simulink model "sauna_sim"  (R2023a)
settings: Solver=VariableStepAuto  StartTime=0.0  StopTime=3600*2  RelTol=1e-3  AbsTol=1e-3
undefined symbols (not defined in the file or in its folder): cost_electricity, cost_gas, gebouw2_temp, gebouw_temp, mean_mean, opgiet_deur_d, opgiet_deur_opp, opgiet_muur_1_hout_d, opgiet_muur_1_isol_d, opgiet_muur_1_opp, opgiet_muur_2_opp, opgiet_muur_3_opp, opgiet_muur_4_opp, opgiet_plafond_opp, opgiet_volume, R_hout, R_hout_plafond, R_isol, R_muur_2_gips, R_muur_3_gips, R_muur_3_raam, R_muur_4_buiten, R_muur_4_gips, R_muur_4_raam, R_opgiet_hout, R_opgiet_isol, R_sauna2_deur, R_se, R_si, rho_lucht, sauna1_deur_d, sauna1_deur_opp, sauna1_muur_1_hout_d, sauna1_muur_1_isol_d, sauna1_muur_1_opp, sauna1_muur_2_gips_d, sauna1_muur_2_opp, sauna1_muur_3_gips_d, sauna1_muur_3_opp, sauna1_muur_4_gips_d, sauna1_muur_4_opp, sauna1_plafond_hout_d, sauna1_plafond_isol_d, sauna1_plafond_opp, sauna1_R_muur_2_gips, sauna1_R_muur_3_gips, sauna1_R_muur_4_gips, sauna1_vol, sauna2_deur_opp, sauna2_muur_1_hout_d, sauna2_muur_1_isol_d, sauna2_muur_1_opp, sauna2_muur_2_gips_d, sauna2_muur_2_opp, sauna2_muur_3_gips_d, sauna2_muur_3_opp, sauna2_muur_3_raam_d, sauna2_muur_3_raam_opp, sauna2_muur_4_gips_d, sauna2_muur_4_opp ... (+6)
libraries: fl_lib x491, nesl_utility x30
(part 1 of 6)
settings Model: Creator=thoma  LastModifiedBy=thoma
settings SolverCC: AutoScaleAbsTol=off  AlgebraicLoopSolver=TrustRegion  MaxZcPerStep=1
settings DebuggingCC: UnconnectedInputMsg=warning  UnconnectedOutputMsg=warning  UnconnectedLineMsg=warning  SymbolicDimsDataTypeCodeGenerationDiagnostic=none
settings ModelReferenceCC: EnableRefExpFcnMdlSchedulingChecks=on
settings SFSimCC: CustomCodeUndefinedFunction=UseInterfaceOnly
settings RTWCC: DLArmComputeVersion=19.05
settings SimscapeCC: SimscapeLogType=all  SimscapeLogSimulationStatistics=on  SimscapeLogDataHistory=10000

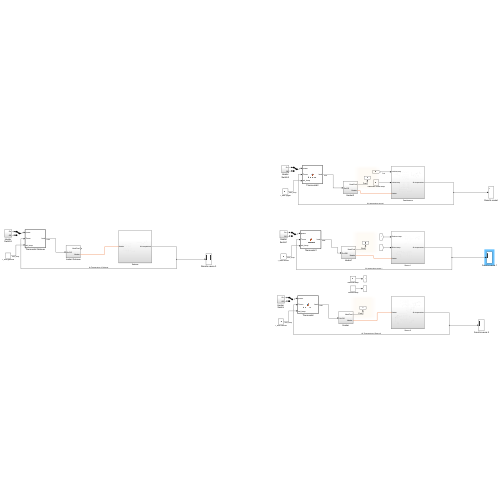
[thumbnail: Simulink's stored preview of the top-level diagram]
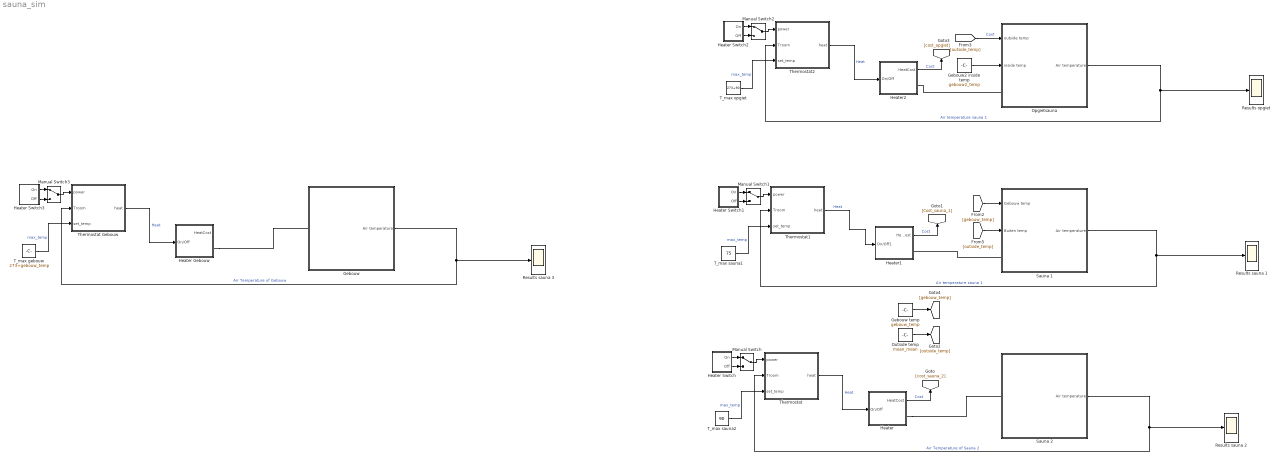
== system sauna_sim ==
  Gebouw : Subsystem
  Gebouw temp : Constant  Value=gebouw_temp
  Gebouw2 inside temp : Constant  Value=gebouw2_temp
  Heater : Subsystem
  Heater Switch : Subsystem
  Heater Switch1 : Subsystem
  Heater Switch2 : Subsystem
  Heater Switch3 : Subsystem
  Heater Gebouw : Subsystem
  Heater1 : Subsystem
  Heater2 : Subsystem
  Manual Switch{,1..3} (4 alike) : ManualSwitch
  Opgietsauna : Subsystem
  Outside temp : Constant  Value=mean_mean
  Results opgiet : Scope
  Results sauna 1 : Scope
  Results sauna 2 : Scope
  Results sauna 3 : Scope
  Sauna 1 : Subsystem
  Sauna 2 : Subsystem
  T_max gebouw : Constant  Value=273+gebouw_temp
  T_max opgiet : Constant  Value=273+90
  T_max sauna1 : Constant  Value=75
  T_max sauna2 : Constant  Value=90
  Thermostat : MATLAB Function  TreatAsAtomicUnit=on
  Thermostat Gebouw : MATLAB Function  TreatAsAtomicUnit=on
  Thermostat1 : MATLAB Function  TreatAsAtomicUnit=on
  Thermostat2 : MATLAB Function  TreatAsAtomicUnit=on
  wires:
  Manual Switch/1 -> Thermostat/1(power)
  Heater Switch/1(On) -> Manual Switch/1
  Heater Switch/2(Off) -> Manual Switch/2
  Thermostat/1(heat) -> Heater/1(On/Off)  "Heat"
  Sauna 2/1(Air temperature) -> Results sauna 2/1, Thermostat/2(Troom)  "Air Temperature of Sauna 2"
  Heater/1(HeatCost) -> [cost_sauna_2]  "Cost"
  T_max sauna2/1 -> Thermostat/3(set_temp)  "max_temp"
  Heater Switch1/1(On) -> Manual Switch1/1
  Heater Switch1/2(Off) -> Manual Switch1/2
  Manual Switch1/1 -> Thermostat1/1(power)
  T_max sauna1/1 -> Thermostat1/3(set_temp)  "max_temp"
  Thermostat1/1(heat) -> Heater1/1(On/Off1)  "Heat"
  Heater1/1(HeatCost) -> [Cost_sauna_1]  "Cost"
  Sauna 1/1(Air temperature) -> Thermostat1/2(Troom), Results sauna 1/1  "Air temperature sauna 1"
  Gebouw2 inside temp/1 -> Opgietsauna/2(inside temp)
  Outside temp/1 -> [outside_temp]
  [outside_temp] -> Opgietsauna/1(outside temp)  "Cost"
  T_max opgiet/1 -> Thermostat2/3(set_temp)  "max_temp"
  Heater2/1(HeatCost) -> [cost_opgiet]  "Cost"
  Manual Switch2/1 -> Thermostat2/1(power)
  Thermostat2/1(heat) -> Heater2/1(On/Off)  "Heat"
  Opgietsauna/1(Air temperature) -> Thermostat2/2(Troom), Results opgiet/1  "Air temperature sauna 1"
  Heater Switch2/1(On) -> Manual Switch2/1
  Heater Switch2/2(Off) -> Manual Switch2/2
  Gebouw temp/1 -> [gebouw_temp]
  [gebouw_temp] -> Sauna 1/1(Gebouw temp)
  [outside_temp] -> Sauna 1/2(Buiten temp)
  Thermostat Gebouw/1(heat) -> Heater Gebouw/1(On/Off)  "Heat"
  Heater Switch3/1(On) -> Manual Switch3/1
  T_max gebouw/1 -> Thermostat Gebouw/3(set_temp)  "max_temp"
  Gebouw/1(Air temperature) -> Results sauna 3/1, Thermostat Gebouw/2(Troom)  "Air Temperature of Gebouw"
  Heater Switch3/2(Off) -> Manual Switch3/2
  Manual Switch3/1 -> Thermostat Gebouw/1(power)
  connections:
  Sauna 1/LConn1 -- Heater1/RConn1
  Opgietsauna/LConn1 -- Heater2/RConn1
  Heater/RConn1 -- Sauna 2/LConn1
  Heater Gebouw/RConn1 -- Gebouw/LConn1

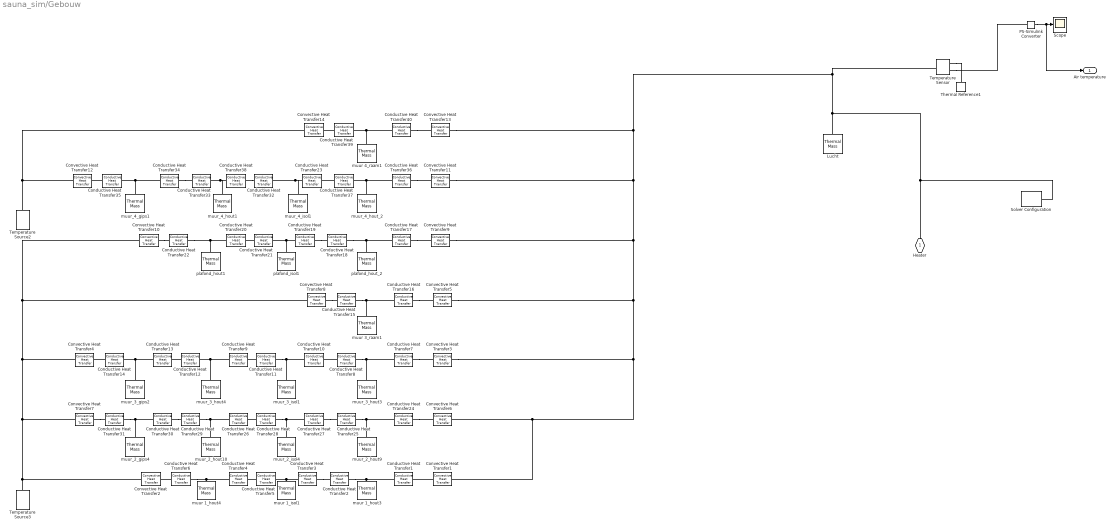
== system sauna_sim/Gebouw ==
  Conductive Heat Transfer{1..2,4,6} (4 alike) : fl_lib/Thermal/Thermal Elements/Conductive Heat Transfer  thermal_type=foundation.enum.ConstantVariableTabulated.Constant  wall_geometry=foundation.enum.ConductionWallGeometry.Planar  area=sauna2_muur_1_opp m^2  thickness=sauna2_muur_1_hout_d/2 m  d_in=0.05 m  d_out=0.1 m  L=1 m  th_cond_min=10 W/(K*m)  th_cond=l_poplar W/(K*m)  th_cond_TLU=[413, 401, 392, 383, 371, 357, 342] W/(K*m)  temp_TLU=[200, 273, 400, 600, 800, 1000, 1200] K  T_specify=off  T_priority=None  T=0 K  T_nominal_specify=off  T_nominal_unit=K  T_nominal_value=1  Q_specify=off  Q_priority=None  Q=0 W  Q_nominal_specify=off  Q_nominal_unit=W  Q_nominal_value=1
  Conductive Heat Transfer10 : fl_lib/Thermal/Thermal Elements/Conductive Heat Transfer  thermal_type=foundation.enum.ConstantVariableTabulated.Constant  wall_geometry=foundation.enum.ConductionWallGeometry.Planar  area=sauna2_muur_3_opp m^2  thickness=sauna2_muur_1_isol_d/2 m  d_in=0.05 m  d_out=0.1 m  L=1 m  th_cond_min=10 W/(K*m)  th_cond=l_isol W/(K*m)  th_cond_TLU=[413, 401, 392, 383, 371, 357, 342] W/(K*m)  temp_TLU=[200, 273, 400, 600, 800, 1000, 1200] K  T_specify=off  T_priority=None  T=0 K  T_nominal_specify=off  T_nominal_unit=K  T_nominal_value=1  Q_specify=off  Q_priority=None  Q=0 W  Q_nominal_specify=off  Q_nominal_unit=W  Q_nominal_value=1
  Conductive Heat Transfer11 : fl_lib/Thermal/Thermal Elements/Conductive Heat Transfer  thermal_type=foundation.enum.ConstantVariableTabulated.Constant  wall_geometry=foundation.enum.ConductionWallGeometry.Planar  area=sauna2_muur_3_opp m^2  thickness=sauna2_muur_1_isol_d/2 m  d_in=0.05 m  d_out=0.1 m  L=1 m  th_cond_min=10 W/(K*m)  th_cond=l_isol W/(K*m)  th_cond_TLU=[413, 401, 392, 383, 371, 357, 342] W/(K*m)  temp_TLU=[200, 273, 400, 600, 800, 1000, 1200] K  T_specify=off  T_priority=None  T=0 K  T_nominal_specify=off  T_nominal_unit=K  T_nominal_value=1  Q_specify=off  Q_priority=None  Q=0 W  Q_nominal_specify=off  Q_nominal_unit=W  Q_nominal_value=1
  Conductive Heat Transfer{7..9,12} (4 alike) : fl_lib/Thermal/Thermal Elements/Conductive Heat Transfer  thermal_type=foundation.enum.ConstantVariableTabulated.Constant  wall_geometry=foundation.enum.ConductionWallGeometry.Planar  area=sauna2_muur_3_opp m^2  thickness=sauna2_muur_1_hout_d/2 m  d_in=0.05 m  d_out=0.1 m  L=1 m  th_cond_min=10 W/(K*m)  th_cond=l_poplar W/(K*m)  th_cond_TLU=[413, 401, 392, 383, 371, 357, 342] W/(K*m)  temp_TLU=[200, 273, 400, 600, 800, 1000, 1200] K  T_specify=off  T_priority=None  T=0 K  T_nominal_specify=off  T_nominal_unit=K  T_nominal_value=1  Q_specify=off  Q_priority=None  Q=0 W  Q_nominal_specify=off  Q_nominal_unit=W  Q_nominal_value=1
  Conductive Heat Transfer13 : fl_lib/Thermal/Thermal Elements/Conductive Heat Transfer  thermal_type=foundation.enum.ConstantVariableTabulated.Constant  wall_geometry=foundation.enum.ConductionWallGeometry.Planar  area=sauna2_muur_3_opp m^2  thickness=sauna2_muur_3_gips_d/2 m  d_in=0.05 m  d_out=0.1 m  L=1 m  th_cond_min=10 W/(K*m)  th_cond=l_gips W/(K*m)  th_cond_TLU=[413, 401, 392, 383, 371, 357, 342] W/(K*m)  temp_TLU=[200, 273, 400, 600, 800, 1000, 1200] K  T_specify=off  T_priority=None  T=0 K  T_nominal_specify=off  T_nominal_unit=K  T_nominal_value=1  Q_specify=off  Q_priority=None  Q=0 W  Q_nominal_specify=off  Q_nominal_unit=W  Q_nominal_value=1
  Conductive Heat Transfer14 : fl_lib/Thermal/Thermal Elements/Conductive Heat Transfer  thermal_type=foundation.enum.ConstantVariableTabulated.Constant  wall_geometry=foundation.enum.ConductionWallGeometry.Planar  area=sauna2_muur_3_opp m^2  thickness=sauna2_muur_3_gips_d/2 m  d_in=0.05 m  d_out=0.1 m  L=1 m  th_cond_min=10 W/(K*m)  th_cond=l_gips W/(K*m)  th_cond_TLU=[413, 401, 392, 383, 371, 357, 342] W/(K*m)  temp_TLU=[200, 273, 400, 600, 800, 1000, 1200] K  T_specify=off  T_priority=None  T=0 K  T_nominal_specify=off  T_nominal_unit=K  T_nominal_value=1  Q_specify=off  Q_priority=None  Q=0 W  Q_nominal_specify=off  Q_nominal_unit=W  Q_nominal_value=1
  Conductive Heat Transfer15 : fl_lib/Thermal/Thermal Elements/Conductive Heat Transfer  thermal_type=foundation.enum.ConstantVariableTabulated.Constant  wall_geometry=foundation.enum.ConductionWallGeometry.Planar  area=sauna2_muur_3_raam_opp m^2  thickness=sauna2_muur_3_raam_d/2 m  d_in=0.05 m  d_out=0.1 m  L=1 m  th_cond_min=10 W/(K*m)  th_cond=l_glas W/(K*m)  th_cond_TLU=[413, 401, 392, 383, 371, 357, 342] W/(K*m)  temp_TLU=[200, 273, 400, 600, 800, 1000, 1200] K  T_specify=off  T_priority=None  T=0 K  T_nominal_specify=off  T_nominal_unit=K  T_nominal_value=1  Q_specify=off  Q_priority=None  Q=0 W  Q_nominal_specify=off  Q_nominal_unit=W  Q_nominal_value=1
  Conductive Heat Transfer16 : fl_lib/Thermal/Thermal Elements/Conductive Heat Transfer  thermal_type=foundation.enum.ConstantVariableTabulated.Constant  wall_geometry=foundation.enum.ConductionWallGeometry.Planar  area=sauna2_muur_3_raam_opp m^2  thickness=sauna2_muur_3_raam_d/2 m  d_in=0.05 m  d_out=0.1 m  L=1 m  th_cond_min=10 W/(K*m)  th_cond=l_glas W/(K*m)  th_cond_TLU=[413, 401, 392, 383, 371, 357, 342] W/(K*m)  temp_TLU=[200, 273, 400, 600, 800, 1000, 1200] K  T_specify=off  T_priority=None  T=0 K  T_nominal_specify=off  T_nominal_unit=K  T_nominal_value=1  Q_specify=off  Q_priority=None  Q=0 W  Q_nominal_specify=off  Q_nominal_unit=W  Q_nominal_value=1
  Conductive Heat Transfer{17..18,20,22} (4 alike) : fl_lib/Thermal/Thermal Elements/Conductive Heat Transfer  thermal_type=foundation.enum.ConstantVariableTabulated.Constant  wall_geometry=foundation.enum.ConductionWallGeometry.Planar  area=sauna2_plafond_opp m^2  thickness=sauna2_plafond_hout_d/2 m  d_in=0.05 m  d_out=0.1 m  L=1 m  th_cond_min=10 W/(K*m)  th_cond=l_poplar W/(K*m)  th_cond_TLU=[413, 401, 392, 383, 371, 357, 342] W/(K*m)  temp_TLU=[200, 273, 400, 600, 800, 1000, 1200] K  T_specify=off  T_priority=None  T=0 K  T_nominal_specify=off  T_nominal_unit=K  T_nominal_value=1  Q_specify=off  Q_priority=None  Q=0 W  Q_nominal_specify=off  Q_nominal_unit=W  Q_nominal_value=1
  Conductive Heat Transfer19 : fl_lib/Thermal/Thermal Elements/Conductive Heat Transfer  thermal_type=foundation.enum.ConstantVariableTabulated.Constant  wall_geometry=foundation.enum.ConductionWallGeometry.Planar  area=sauna2_plafond_opp m^2  thickness=sauna2_plafond_isol_d/2 m  d_in=0.05 m  d_out=0.1 m  L=1 m  th_cond_min=10 W/(K*m)  th_cond=l_isol W/(K*m)  th_cond_TLU=[413, 401, 392, 383, 371, 357, 342] W/(K*m)  temp_TLU=[200, 273, 400, 600, 800, 1000, 1200] K  T_specify=off  T_priority=None  T=0 K  T_nominal_specify=off  T_nominal_unit=K  T_nominal_value=1  Q_specify=off  Q_priority=None  Q=0 W  Q_nominal_specify=off  Q_nominal_unit=W  Q_nominal_value=1
  Conductive Heat Transfer21 : fl_lib/Thermal/Thermal Elements/Conductive Heat Transfer  thermal_type=foundation.enum.ConstantVariableTabulated.Constant  wall_geometry=foundation.enum.ConductionWallGeometry.Planar  area=sauna2_plafond_opp m^2  thickness=sauna2_plafond_isol_d/2 m  d_in=0.05 m  d_out=0.1 m  L=1 m  th_cond_min=10 W/(K*m)  th_cond=l_isol W/(K*m)  th_cond_TLU=[413, 401, 392, 383, 371, 357, 342] W/(K*m)  temp_TLU=[200, 273, 400, 600, 800, 1000, 1200] K  T_specify=off  T_priority=None  T=0 K  T_nominal_specify=off  T_nominal_unit=K  T_nominal_value=1  Q_specify=off  Q_priority=None  Q=0 W  Q_nominal_specify=off  Q_nominal_unit=W  Q_nominal_value=1
  Conductive Heat Transfer23 : fl_lib/Thermal/Thermal Elements/Conductive Heat Transfer  thermal_type=foundation.enum.ConstantVariableTabulated.Constant  wall_geometry=foundation.enum.ConductionWallGeometry.Planar  area=sauna2_muur_4_opp m^2  thickness=sauna2_muur_1_isol_d/2 m  d_in=0.05 m  d_out=0.1 m  L=1 m  th_cond_min=10 W/(K*m)  th_cond=l_isol W/(K*m)  th_cond_TLU=[413, 401, 392, 383, 371, 357, 342] W/(K*m)  temp_TLU=[200, 273, 400, 600, 800, 1000, 1200] K  T_specify=off  T_priority=None  T=0 K  T_nominal_specify=off  T_nominal_unit=K  T_nominal_value=1  Q_specify=off  Q_priority=None  Q=0 W  Q_nominal_specify=off  Q_nominal_unit=W  Q_nominal_value=1
  Conductive Heat Transfer{24..26,29} (4 alike) : fl_lib/Thermal/Thermal Elements/Conductive Heat Transfer  thermal_type=foundation.enum.ConstantVariableTabulated.Constant  wall_geometry=foundation.enum.ConductionWallGeometry.Planar  area=sauna2_muur_2_opp m^2  thickness=sauna2_muur_1_hout_d/2 m  d_in=0.05 m  d_out=0.1 m  L=1 m  th_cond_min=10 W/(K*m)  th_cond=l_poplar W/(K*m)  th_cond_TLU=[413, 401, 392, 383, 371, 357, 342] W/(K*m)  temp_TLU=[200, 273, 400, 600, 800, 1000, 1200] K  T_specify=off  T_priority=None  T=0 K  T_nominal_specify=off  T_nominal_unit=K  T_nominal_value=1  Q_specify=off  Q_priority=None  Q=0 W  Q_nominal_specify=off  Q_nominal_unit=W  Q_nominal_value=1
  Conductive Heat Transfer27 : fl_lib/Thermal/Thermal Elements/Conductive Heat Transfer  thermal_type=foundation.enum.ConstantVariableTabulated.Constant  wall_geometry=foundation.enum.ConductionWallGeometry.Planar  area=sauna2_muur_2_opp m^2  thickness=sauna2_muur_1_isol_d/2 m  d_in=0.05 m  d_out=0.1 m  L=1 m  th_cond_min=10 W/(K*m)  th_cond=l_isol W/(K*m)  th_cond_TLU=[413, 401, 392, 383, 371, 357, 342] W/(K*m)  temp_TLU=[200, 273, 400, 600, 800, 1000, 1200] K  T_specify=off  T_priority=None  T=0 K  T_nominal_specify=off  T_nominal_unit=K  T_nominal_value=1  Q_specify=off  Q_priority=None  Q=0 W  Q_nominal_specify=off  Q_nominal_unit=W  Q_nominal_value=1
  Conductive Heat Transfer28 : fl_lib/Thermal/Thermal Elements/Conductive Heat Transfer  thermal_type=foundation.enum.ConstantVariableTabulated.Constant  wall_geometry=foundation.enum.ConductionWallGeometry.Planar  area=sauna2_muur_2_opp m^2  thickness=sauna2_muur_1_isol_d/2 m  d_in=0.05 m  d_out=0.1 m  L=1 m  th_cond_min=10 W/(K*m)  th_cond=l_isol W/(K*m)  th_cond_TLU=[413, 401, 392, 383, 371, 357, 342] W/(K*m)  temp_TLU=[200, 273, 400, 600, 800, 1000, 1200] K  T_specify=off  T_priority=None  T=0 K  T_nominal_specify=off  T_nominal_unit=K  T_nominal_value=1  Q_specify=off  Q_priority=None  Q=0 W  Q_nominal_specify=off  Q_nominal_unit=W  Q_nominal_value=1
  Conductive Heat Transfer3 : fl_lib/Thermal/Thermal Elements/Conductive Heat Transfer  thermal_type=foundation.enum.ConstantVariableTabulated.Constant  wall_geometry=foundation.enum.ConductionWallGeometry.Planar  area=sauna2_muur_1_opp m^2  thickness=sauna2_muur_1_isol_d/2 m  d_in=0.05 m  d_out=0.1 m  L=1 m  th_cond_min=10 W/(K*m)  th_cond=l_isol W/(K*m)  th_cond_TLU=[413, 401, 392, 383, 371, 357, 342] W/(K*m)  temp_TLU=[200, 273, 400, 600, 800, 1000, 1200] K  T_specify=off  T_priority=None  T=0 K  T_nominal_specify=off  T_nominal_unit=K  T_nominal_value=1  Q_specify=off  Q_priority=None  Q=0 W  Q_nominal_specify=off  Q_nominal_unit=W  Q_nominal_value=1
  Conductive Heat Transfer30 : fl_lib/Thermal/Thermal Elements/Conductive Heat Transfer  thermal_type=foundation.enum.ConstantVariableTabulated.Constant  wall_geometry=foundation.enum.ConductionWallGeometry.Planar  area=sauna2_muur_2_opp m^2  thickness=sauna2_muur_2_gips_d/2 m  d_in=0.05 m  d_out=0.1 m  L=1 m  th_cond_min=10 W/(K*m)  th_cond=l_gips W/(K*m)  th_cond_TLU=[413, 401, 392, 383, 371, 357, 342] W/(K*m)  temp_TLU=[200, 273, 400, 600, 800, 1000, 1200] K  T_specify=off  T_priority=None  T=0 K  T_nominal_specify=off  T_nominal_unit=K  T_nominal_value=1  Q_specify=off  Q_priority=None  Q=0 W  Q_nominal_specify=off  Q_nominal_unit=W  Q_nominal_value=1
  Conductive Heat Transfer31 : fl_lib/Thermal/Thermal Elements/Conductive Heat Transfer  thermal_type=foundation.enum.ConstantVariableTabulated.Constant  wall_geometry=foundation.enum.ConductionWallGeometry.Planar  area=sauna2_muur_2_opp m^2  thickness=sauna2_muur_2_gips_d/2 m  d_in=0.05 m  d_out=0.1 m  L=1 m  th_cond_min=10 W/(K*m)  th_cond=l_gips W/(K*m)  th_cond_TLU=[413, 401, 392, 383, 371, 357, 342] W/(K*m)  temp_TLU=[200, 273, 400, 600, 800, 1000, 1200] K  T_specify=off  T_priority=None  T=0 K  T_nominal_specify=off  T_nominal_unit=K  T_nominal_value=1  Q_specify=off  Q_priority=None  Q=0 W  Q_nominal_specify=off  Q_nominal_unit=W  Q_nominal_value=1
  Conductive Heat Transfer32 : fl_lib/Thermal/Thermal Elements/Conductive Heat Transfer  thermal_type=foundation.enum.ConstantVariableTabulated.Constant  wall_geometry=foundation.enum.ConductionWallGeometry.Planar  area=sauna2_muur_4_opp m^2  thickness=sauna2_muur_1_isol_d/2 m  d_in=0.05 m  d_out=0.1 m  L=1 m  th_cond_min=10 W/(K*m)  th_cond=l_isol W/(K*m)  th_cond_TLU=[413, 401, 392, 383, 371, 357, 342] W/(K*m)  temp_TLU=[200, 273, 400, 600, 800, 1000, 1200] K  T_specify=off  T_priority=None  T=0 K  T_nominal_specify=off  T_nominal_unit=K  T_nominal_value=1  Q_specify=off  Q_priority=None  Q=0 W  Q_nominal_specify=off  Q_nominal_unit=W  Q_nominal_value=1
  Conductive Heat Transfer{33,36..38} (4 alike) : fl_lib/Thermal/Thermal Elements/Conductive Heat Transfer  thermal_type=foundation.enum.ConstantVariableTabulated.Constant  wall_geometry=foundation.enum.ConductionWallGeometry.Planar  area=sauna2_muur_4_opp m^2  thickness=sauna2_muur_1_hout_d/2 m  d_in=0.05 m  d_out=0.1 m  L=1 m  th_cond_min=10 W/(K*m)  th_cond=l_poplar W/(K*m)  th_cond_TLU=[413, 401, 392, 383, 371, 357, 342] W/(K*m)  temp_TLU=[200, 273, 400, 600, 800, 1000, 1200] K  T_specify=off  T_priority=None  T=0 K  T_nominal_specify=off  T_nominal_unit=K  T_nominal_value=1  Q_specify=off  Q_priority=None  Q=0 W  Q_nominal_specify=off  Q_nominal_unit=W  Q_nominal_value=1
  Conductive Heat Transfer34 : fl_lib/Thermal/Thermal Elements/Conductive Heat Transfer  thermal_type=foundation.enum.ConstantVariableTabulated.Constant  wall_geometry=foundation.enum.ConductionWallGeometry.Planar  area=sauna2_muur_4_opp m^2  thickness=sauna2_muur_4_gips_d/2 m  d_in=0.05 m  d_out=0.1 m  L=1 m  th_cond_min=10 W/(K*m)  th_cond=l_gips W/(K*m)  th_cond_TLU=[413, 401, 392, 383, 371, 357, 342] W/(K*m)  temp_TLU=[200, 273, 400, 600, 800, 1000, 1200] K  T_specify=off  T_priority=None  T=0 K  T_nominal_specify=off  T_nominal_unit=K  T_nominal_value=1  Q_specify=off  Q_priority=None  Q=0 W  Q_nominal_specify=off  Q_nominal_unit=W  Q_nominal_value=1
  Conductive Heat Transfer35 : fl_lib/Thermal/Thermal Elements/Conductive Heat Transfer  thermal_type=foundation.enum.ConstantVariableTabulated.Constant  wall_geometry=foundation.enum.ConductionWallGeometry.Planar  area=sauna2_muur_4_opp m^2  thickness=sauna2_muur_4_gips_d/2 m  d_in=0.05 m  d_out=0.1 m  L=1 m  th_cond_min=10 W/(K*m)  th_cond=l_gips W/(K*m)  th_cond_TLU=[413, 401, 392, 383, 371, 357, 342] W/(K*m)  temp_TLU=[200, 273, 400, 600, 800, 1000, 1200] K  T_specify=off  T_priority=None  T=0 K  T_nominal_specify=off  T_nominal_unit=K  T_nominal_value=1  Q_specify=off  Q_priority=None  Q=0 W  Q_nominal_specify=off  Q_nominal_unit=W  Q_nominal_value=1
  Conductive Heat Transfer39 : fl_lib/Thermal/Thermal Elements/Conductive Heat Transfer  thermal_type=foundation.enum.ConstantVariableTabulated.Constant  wall_geometry=foundation.enum.ConductionWallGeometry.Planar  area=sauna2_muur_4_opp m^2  thickness=sauna2_muur_4_raam_d/2 m  d_in=0.05 m  d_out=0.1 m  L=1 m  th_cond_min=10 W/(K*m)  th_cond=sauna2_muur_4_raam_d/R_muur_4_raam W/(K*m)  th_cond_TLU=[413, 401, 392, 383, 371, 357, 342] W/(K*m)  temp_TLU=[200, 273, 400, 600, 800, 1000, 1200] K  T_specify=off  T_priority=None  T=0 K  T_nominal_specify=off  T_nominal_unit=K  T_nominal_value=1  Q_specify=off  Q_priority=None  Q=0 W  Q_nominal_specify=off  Q_nominal_unit=W  Q_nominal_value=1
  Conductive Heat Transfer40 : fl_lib/Thermal/Thermal Elements/Conductive Heat Transfer  thermal_type=foundation.enum.ConstantVariableTabulated.Constant  wall_geometry=foundation.enum.ConductionWallGeometry.Planar  area=sauna2_muur_4_opp m^2  thickness=sauna2_muur_4_raam_d/2 m  d_in=0.05 m  d_out=0.1 m  L=1 m  th_cond_min=10 W/(K*m)  th_cond=sauna2_muur_4_raam_d/R_muur_4_raam W/(K*m)  th_cond_TLU=[413, 401, 392, 383, 371, 357, 342] W/(K*m)  temp_TLU=[200, 273, 400, 600, 800, 1000, 1200] K  T_specify=off  T_priority=None  T=0 K  T_nominal_specify=off  T_nominal_unit=K  T_nominal_value=1  Q_specify=off  Q_priority=None  Q=0 W  Q_nominal_specify=off  Q_nominal_unit=W  Q_nominal_value=1
  Conductive Heat Transfer5 : fl_lib/Thermal/Thermal Elements/Conductive Heat Transfer  thermal_type=foundation.enum.ConstantVariableTabulated.Constant  wall_geometry=foundation.enum.ConductionWallGeometry.Planar  area=sauna2_muur_1_opp m^2  thickness=sauna2_muur_1_isol_d/2 m  d_in=0.05 m  d_out=0.1 m  L=1 m  th_cond_min=10 W/(K*m)  th_cond=l_isol W/(K*m)  th_cond_TLU=[413, 401, 392, 383, 371, 357, 342] W/(K*m)  temp_TLU=[200, 273, 400, 600, 800, 1000, 1200] K  T_specify=off  T_priority=None  T=0 K  T_nominal_specify=off  T_nominal_unit=K  T_nominal_value=1  Q_specify=off  Q_priority=None  Q=0 W  Q_nominal_specify=off  Q_nominal_unit=W  Q_nominal_value=1
  Convective Heat Transfer1 : fl_lib/Thermal/Thermal Elements/Convective Heat Transfer  thermal_type=foundation.enum.constant_variable.constant  area=sauna2_muur_1_opp m^2  heat_tr_coeff=15 W/(K*m^2)  min_heat_tr_coeff=1e-3 W/(K*m^2)  T_specify=off  T_priority=None  T=0 K  T_nominal_specify=off  T_nominal_unit=K  T_nominal_value=1  Q_specify=off  Q_priority=None  Q=0 W  Q_nominal_specify=off  Q_nominal_unit=W  Q_nominal_value=1
  Convective Heat Transfer10 : fl_lib/Thermal/Thermal Elements/Convective Heat Transfer  thermal_type=foundation.enum.constant_variable.constant  area=sauna2_plafond_opp m^2  heat_tr_coeff=15 W/(K*m^2)  min_heat_tr_coeff=1e-3 W/(K*m^2)  T_specify=off  T_priority=None  T=0 K  T_nominal_specify=off  T_nominal_unit=K  T_nominal_value=1  Q_specify=off  Q_priority=None  Q=0 W  Q_nominal_specify=off  Q_nominal_unit=W  Q_nominal_value=1
  Convective Heat Transfer11 : fl_lib/Thermal/Thermal Elements/Convective Heat Transfer  thermal_type=foundation.enum.constant_variable.constant  area=sauna2_muur_4_opp m^2  heat_tr_coeff=15 W/(K*m^2)  min_heat_tr_coeff=1e-3 W/(K*m^2)  T_specify=off  T_priority=None  T=0 K  T_nominal_specify=off  T_nominal_unit=K  T_nominal_value=1  Q_specify=off  Q_priority=None  Q=0 W  Q_nominal_specify=off  Q_nominal_unit=W  Q_nominal_value=1
  Convective Heat Transfer12 : fl_lib/Thermal/Thermal Elements/Convective Heat Transfer  thermal_type=foundation.enum.constant_variable.constant  area=sauna2_muur_4_opp m^2  heat_tr_coeff=30 W/(K*m^2)  min_heat_tr_coeff=1e-3 W/(K*m^2)  T_specify=off  T_priority=None  T=0 K  T_nominal_specify=off  T_nominal_unit=K  T_nominal_value=1  Q_specify=off  Q_priority=None  Q=0 W  Q_nominal_specify=off  Q_nominal_unit=W  Q_nominal_value=1
  Convective Heat Transfer13 : fl_lib/Thermal/Thermal Elements/Convective Heat Transfer  thermal_type=foundation.enum.constant_variable.constant  area=sauna2_muur_4_opp m^2  heat_tr_coeff=15 W/(K*m^2)  min_heat_tr_coeff=1e-3 W/(K*m^2)  T_specify=off  T_priority=None  T=0 K  T_nominal_specify=off  T_nominal_unit=K  T_nominal_value=1  Q_specify=off  Q_priority=None  Q=0 W  Q_nominal_specify=off  Q_nominal_unit=W  Q_nominal_value=1
  Convective Heat Transfer14 : fl_lib/Thermal/Thermal Elements/Convective Heat Transfer  thermal_type=foundation.enum.constant_variable.constant  area=sauna2_muur_4_opp m^2  heat_tr_coeff=30 W/(K*m^2)  min_heat_tr_coeff=1e-3 W/(K*m^2)  T_specify=off  T_priority=None  T=0 K  T_nominal_specify=off  T_nominal_unit=K  T_nominal_value=1  Q_specify=off  Q_priority=None  Q=0 W  Q_nominal_specify=off  Q_nominal_unit=W  Q_nominal_value=1
  Convective Heat Transfer2 : fl_lib/Thermal/Thermal Elements/Convective Heat Transfer  thermal_type=foundation.enum.constant_variable.constant  area=sauna2_muur_1_opp m^2  heat_tr_coeff=15 W/(K*m^2)  min_heat_tr_coeff=1e-3 W/(K*m^2)  T_specify=off  T_priority=None  T=0 K  T_nominal_specify=off  T_nominal_unit=K  T_nominal_value=1  Q_specify=off  Q_priority=None  Q=0 W  Q_nominal_specify=off  Q_nominal_unit=W  Q_nominal_value=1
  Convective Heat Transfer3 : fl_lib/Thermal/Thermal Elements/Convective Heat Transfer  thermal_type=foundation.enum.constant_variable.constant  area=sauna2_muur_3_opp m^2  heat_tr_coeff=15 W/(K*m^2)  min_heat_tr_coeff=1e-3 W/(K*m^2)  T_specify=off  T_priority=None  T=0 K  T_nominal_specify=off  T_nominal_unit=K  T_nominal_value=1  Q_specify=off  Q_priority=None  Q=0 W  Q_nominal_specify=off  Q_nominal_unit=W  Q_nominal_value=1
  Convective Heat Transfer4 : fl_lib/Thermal/Thermal Elements/Convective Heat Transfer  thermal_type=foundation.enum.constant_variable.constant  area=sauna2_muur_3_opp m^2  heat_tr_coeff=15 W/(K*m^2)  min_heat_tr_coeff=1e-3 W/(K*m^2)  T_specify=off  T_priority=None  T=0 K  T_nominal_specify=off  T_nominal_unit=K  T_nominal_value=1  Q_specify=off  Q_priority=None  Q=0 W  Q_nominal_specify=off  Q_nominal_unit=W  Q_nominal_value=1
  Convective Heat Transfer5 : fl_lib/Thermal/Thermal Elements/Convective Heat Transfer  thermal_type=foundation.enum.constant_variable.constant  area=sauna2_muur_3_raam_opp m^2  heat_tr_coeff=15 W/(K*m^2)  min_heat_tr_coeff=1e-3 W/(K*m^2)  T_specify=off  T_priority=None  T=0 K  T_nominal_specify=off  T_nominal_unit=K  T_nominal_value=1  Q_specify=off  Q_priority=None  Q=0 W  Q_nominal_specify=off  Q_nominal_unit=W  Q_nominal_value=1
  Convective Heat Transfer6 : fl_lib/Thermal/Thermal Elements/Convective Heat Transfer  thermal_type=foundation.enum.constant_variable.constant  area=sauna2_muur_2_opp m^2  heat_tr_coeff=15 W/(K*m^2)  min_heat_tr_coeff=1e-3 W/(K*m^2)  T_specify=off  T_priority=None  T=0 K  T_nominal_specify=off  T_nominal_unit=K  T_nominal_value=1  Q_specify=off  Q_priority=None  Q=0 W  Q_nominal_specify=off  Q_nominal_unit=W  Q_nominal_value=1
  Convective Heat Transfer7 : fl_lib/Thermal/Thermal Elements/Convective Heat Transfer  thermal_type=foundation.enum.constant_variable.constant  area=sauna2_muur_2_opp m^2  heat_tr_coeff=15 W/(K*m^2)  min_heat_tr_coeff=1e-3 W/(K*m^2)  T_specify=off  T_priority=None  T=0 K  T_nominal_specify=off  T_nominal_unit=K  T_nominal_value=1  Q_specify=off  Q_priority=None  Q=0 W  Q_nominal_specify=off  Q_nominal_unit=W  Q_nominal_value=1
  Convective Heat Transfer8 : fl_lib/Thermal/Thermal Elements/Convective Heat Transfer  thermal_type=foundation.enum.constant_variable.constant  area=sauna2_muur_3_raam_opp m^2  heat_tr_coeff=15 W/(K*m^2)  min_heat_tr_coeff=1e-3 W/(K*m^2)  T_specify=off  T_priority=None  T=0 K  T_nominal_specify=off  T_nominal_unit=K  T_nominal_value=1  Q_specify=off  Q_priority=None  Q=0 W  Q_nominal_specify=off  Q_nominal_unit=W  Q_nominal_value=1
  Convective Heat Transfer9 : fl_lib/Thermal/Thermal Elements/Convective Heat Transfer  thermal_type=foundation.enum.constant_variable.constant  area=sauna2_plafond_opp m^2  heat_tr_coeff=15 W/(K*m^2)  min_heat_tr_coeff=1e-3 W/(K*m^2)  T_specify=off  T_priority=None  T=0 K  T_nominal_specify=off  T_nominal_unit=K  T_nominal_value=1  Q_specify=off  Q_priority=None  Q=0 W  Q_nominal_specify=off  Q_nominal_unit=W  Q_nominal_value=1
  Lucht : fl_lib/Thermal/Thermal Elements/Thermal Mass  mass_type=foundation.enum.constant_variable.constant  mass=sauna2_vol*rho_lucht kg  sp_heat=cp_lucht J/(K*kg)  mass_min=1e-6 kg  num_ports=foundation.enum.numPorts2.one  m_specify=off  m_priority=High  m=1 kg  m_nominal_specify=off  m_nominal_unit=kg  m_nominal_value=1  T_specify=on  T_priority=High  T=300 K  T_nominal_specify=off  T_nominal_unit=K  T_nominal_value=1  Q_specify=off  Q_priority=None  Q=0 W  Q_nominal_specify=off  Q_nominal_unit=W  Q_nominal_value=1
  PS-Simulink Converter : nesl_utility/PS-Simulink Converter  PhysicalDomain=network_engine_domain  SubClassName=ps_output  LeftPortType=input  RightPortType=output  PseudoPeriodic=off  Frequencies=[]  VectorFormat=1-D array  Unit=degC  AffineConversion=on
  Scope : Scope
  Solver Configuration : nesl_utility/Solver Configuration  PhysicalDomain=network_engine_domain  SubClassName=solver  LeftPortType=input  RightPortType=generic  Tones=[]  Harmonics=[]  SimulateNoise=off  Profile=off  UseLocalSampling=off  EnableSwitchedLinearOptims=on  FrequencyDomain=off  UseCCode=off  RelTol=0.001  AbsTol=1e-06  MinStep=1e-09  ToWorkspace=off  RevertToSquareIcSolve=off  NumHomotopyIterations=100  PhasorMode=off  PhasorModeNumHarmonics=1  ConsistencySolver=NEWTON_XTOL_AFTER_FTOL  IndexReductionMethod=DerivativeReplacement  DoDC=off  ResidualTolerance=1e-09  ConsistencyTolSource=GLOBAL  ConsistencyAbsTol=0.001  ConsistencyRelTol=0.001  ConsistencyTolFactor=0.001  UseLocalSolver=off  LocalSolverChoice=NE_BACKWARD_EULER_ADVANCER  ResolveIndetEquations=on  FunctionEvalNumThread=1  LocalSolverSampleTime=0.001  DoFixedCost=off  MaxNonlinIter=3  MaxModeIter=2  ComputeImpulses=off  ImpulseIterations=2  LinearAlgebra=auto  LinearAlgebraNumThread=0  EquationFormulation=NE_TIME_EF  DelaysMemoryBudget=1024  AutomaticFiltering=on  FilteringTimeConstant=0.001  PartitionStorageMethod=AS_NEEDED  PartitionMemoryBudget=1024  PartitionMethod=ROBUST
  Temperature Sensor : fl_lib/Thermal/Thermal Sensors/Temperature Sensor  temperature_measure=foundation.enum.MeasurementReference.difference
  Temperature Source2 : fl_lib/Thermal/Thermal Sources/Temperature Source  temperature=mean_mean+273 K
  Temperature Source3 : fl_lib/Thermal/Thermal Sources/Temperature Source  temperature=gebouw_temp+273 K
  Thermal Reference1 : fl_lib/Thermal/Thermal Elements/Thermal Reference
  muur 1_hout3 : fl_lib/Thermal/Thermal Elements/Thermal Mass  mass_type=foundation.enum.constant_variable.constant  mass=sauna2_muur_1_hout_1_m kg  sp_heat=cp_poplar J/(K*kg)  mass_min=1e-6 kg  num_ports=foundation.enum.numPorts2.one  m_specify=off  m_priority=High  m=1 kg  m_nominal_specify=off  m_nominal_unit=kg  m_nominal_value=1  T_specify=off  T_priority=High  T=300 K  T_nominal_specify=off  T_nominal_unit=K  T_nominal_value=1  Q_specify=off  Q_priority=None  Q=0 W  Q_nominal_specify=off  Q_nominal_unit=W  Q_nominal_value=1
  muur 1_hout4 : fl_lib/Thermal/Thermal Elements/Thermal Mass  mass_type=foundation.enum.constant_variable.constant  mass=sauna2_muur_1_hout_2_m kg  sp_heat=cp_poplar J/(K*kg)  mass_min=1e-6 kg  num_ports=foundation.enum.numPorts2.one  m_specify=off  m_priority=High  m=1 kg  m_nominal_specify=off  m_nominal_unit=kg  m_nominal_value=1  T_specify=off  T_priority=High  T=300 K  T_nominal_specify=off  T_nominal_unit=K  T_nominal_value=1  Q_specify=off  Q_priority=None  Q=0 W  Q_nominal_specify=off  Q_nominal_unit=W  Q_nominal_value=1
  muur 1_isol1 : fl_lib/Thermal/Thermal Elements/Thermal Mass  mass_type=foundation.enum.constant_variable.constant  mass=sauna2_muur_1_isol_m kg  sp_heat=cp_isol J/(K*kg)  mass_min=1e-6 kg  num_ports=foundation.enum.numPorts2.one  m_specify=off  m_priority=High  m=1 kg  m_nominal_specify=off  m_nominal_unit=kg  m_nominal_value=1  T_specify=off  T_priority=High  T=300 K  T_nominal_specify=off  T_nominal_unit=K  T_nominal_value=1  Q_specify=off  Q_priority=None  Q=0 W  Q_nominal_specify=off  Q_nominal_unit=W  Q_nominal_value=1
  muur 3_raam1 : fl_lib/Thermal/Thermal Elements/Thermal Mass  mass_type=foundation.enum.constant_variable.constant  mass=sauna2_muur_3_raam_m kg  sp_heat=cp_glas J/(K*kg)  mass_min=1e-6 kg  num_ports=foundation.enum.numPorts2.one  m_specify=off  m_priority=High  m=1 kg  m_nominal_specify=off  m_nominal_unit=kg  m_nominal_value=1  T_specify=off  T_priority=High  T=300 K  T_nominal_specify=off  T_nominal_unit=K  T_nominal_value=1  Q_specify=off  Q_priority=None  Q=0 W  Q_nominal_specify=off  Q_nominal_unit=W  Q_nominal_value=1
  muur 4_raam1 : fl_lib/Thermal/Thermal Elements/Thermal Mass  mass_type=foundation.enum.constant_variable.constant  mass=sauna2_muur_4_raam_m kg  sp_heat=cp_glas J/(K*kg)  mass_min=1e-6 kg  num_ports=foundation.enum.numPorts2.one  m_specify=off  m_priority=High  m=1 kg  m_nominal_specify=off  m_nominal_unit=kg  m_nominal_value=1  T_specify=off  T_priority=High  T=300 K  T_nominal_specify=off  T_nominal_unit=K  T_nominal_value=1  Q_specify=off  Q_priority=None  Q=0 W  Q_nominal_specify=off  Q_nominal_unit=W  Q_nominal_value=1
  muur_2_gips4 : fl_lib/Thermal/Thermal Elements/Thermal Mass  mass_type=foundation.enum.constant_variable.constant  mass=sauna2_muur_2_gips_m kg  sp_heat=cp_gips J/(K*kg)  mass_min=1e-6 kg  num_ports=foundation.enum.numPorts2.one  m_specify=off  m_priority=High  m=1 kg  m_nominal_specify=off  m_nominal_unit=kg  m_nominal_value=1  T_specify=off  T_priority=High  T=300 K  T_nominal_specify=off  T_nominal_unit=K  T_nominal_value=1  Q_specify=off  Q_priority=None  Q=0 W  Q_nominal_specify=off  Q_nominal_unit=W  Q_nominal_value=1
  muur_2_hout10 : fl_lib/Thermal/Thermal Elements/Thermal Mass  mass_type=foundation.enum.constant_variable.constant  mass=sauna2_muur_2_hout_1_m kg  sp_heat=cp_poplar J/(K*kg)  mass_min=1e-6 kg  num_ports=foundation.enum.numPorts2.one  m_specify=off  m_priority=High  m=1 kg  m_nominal_specify=off  m_nominal_unit=kg  m_nominal_value=1  T_specify=off  T_priority=High  T=300 K  T_nominal_specify=off  T_nominal_unit=K  T_nominal_value=1  Q_specify=off  Q_priority=None  Q=0 W  Q_nominal_specify=off  Q_nominal_unit=W  Q_nominal_value=1
  muur_2_hout9 : fl_lib/Thermal/Thermal Elements/Thermal Mass  mass_type=foundation.enum.constant_variable.constant  mass=sauna2_muur_2_hout_1_m kg  sp_heat=cp_poplar J/(K*kg)  mass_min=1e-6 kg  num_ports=foundation.enum.numPorts2.one  m_specify=off  m_priority=High  m=1 kg  m_nominal_specify=off  m_nominal_unit=kg  m_nominal_value=1  T_specify=off  T_priority=High  T=300 K  T_nominal_specify=off  T_nominal_unit=K  T_nominal_value=1  Q_specify=off  Q_priority=None  Q=0 W  Q_nominal_specify=off  Q_nominal_unit=W  Q_nominal_value=1
  muur_2_isol4 : fl_lib/Thermal/Thermal Elements/Thermal Mass  mass_type=foundation.enum.constant_variable.constant  mass=sauna2_muur_2_isol_m kg  sp_heat=cp_isol J/(K*kg)  mass_min=1e-6 kg  num_ports=foundation.enum.numPorts2.one  m_specify=off  m_priority=High  m=1 kg  m_nominal_specify=off  m_nominal_unit=kg  m_nominal_value=1  T_specify=off  T_priority=High  T=300 K  T_nominal_specify=off  T_nominal_unit=K  T_nominal_value=1  Q_specify=off  Q_priority=None  Q=0 W  Q_nominal_specify=off  Q_nominal_unit=W  Q_nominal_value=1
  muur_3_gips2 : fl_lib/Thermal/Thermal Elements/Thermal Mass  mass_type=foundation.enum.constant_variable.constant  mass=sauna2_muur_3_gips_m kg  sp_heat=cp_gips J/(K*kg)  mass_min=1e-6 kg  num_ports=foundation.enum.numPorts2.one  m_specify=off  m_priority=High  m=1 kg  m_nominal_specify=off  m_nominal_unit=kg  m_nominal_value=1  T_specify=off  T_priority=High  T=300 K  T_nominal_specify=off  T_nominal_unit=K  T_nominal_value=1  Q_specify=off  Q_priority=None  Q=0 W  Q_nominal_specify=off  Q_nominal_unit=W  Q_nominal_value=1
  muur_3_hout3 : fl_lib/Thermal/Thermal Elements/Thermal Mass  mass_type=foundation.enum.constant_variable.constant  mass=sauna2_muur_3_hout_1_m kg  sp_heat=cp_poplar J/(K*kg)  mass_min=1e-6 kg  num_ports=foundation.enum.numPorts2.one  m_specify=off  m_priority=High  m=1 kg  m_nominal_specify=off  m_nominal_unit=kg  m_nominal_value=1  T_specify=off  T_priority=High  T=300 K  T_nominal_specify=off  T_nominal_unit=K  T_nominal_value=1  Q_specify=off  Q_priority=None  Q=0 W  Q_nominal_specify=off  Q_nominal_unit=W  Q_nominal_value=1
  muur_3_hout4 : fl_lib/Thermal/Thermal Elements/Thermal Mass  mass_type=foundation.enum.constant_variable.constant  mass=sauna2_muur_3_hout_2_m kg  sp_heat=cp_poplar J/(K*kg)  mass_min=1e-6 kg  num_ports=foundation.enum.numPorts2.one  m_specify=off  m_priority=High  m=1 kg  m_nominal_specify=off  m_nominal_unit=kg  m_nominal_value=1  T_specify=off  T_priority=High  T=300 K  T_nominal_specify=off  T_nominal_unit=K  T_nominal_value=1  Q_specify=off  Q_priority=None  Q=0 W  Q_nominal_specify=off  Q_nominal_unit=W  Q_nominal_value=1
  muur_3_isol1 : fl_lib/Thermal/Thermal Elements/Thermal Mass  mass_type=foundation.enum.constant_variable.constant  mass=sauna2_muur_3_isol_m kg  sp_heat=cp_isol J/(K*kg)  mass_min=1e-6 kg  num_ports=foundation.enum.numPorts2.one  m_specify=off  m_priority=High  m=1 kg  m_nominal_specify=off  m_nominal_unit=kg  m_nominal_value=1  T_specify=off  T_priority=High  T=300 K  T_nominal_specify=off  T_nominal_unit=K  T_nominal_value=1  Q_specify=off  Q_priority=None  Q=0 W  Q_nominal_specify=off  Q_nominal_unit=W  Q_nominal_value=1
  muur_4_gips1 : fl_lib/Thermal/Thermal Elements/Thermal Mass  mass_type=foundation.enum.constant_variable.constant  mass=sauna2_muur_4_gips_m kg  sp_heat=cp_gips J/(K*kg)  mass_min=1e-6 kg  num_ports=foundation.enum.numPorts2.one  m_specify=off  m_priority=High  m=1 kg  m_nominal_specify=off  m_nominal_unit=kg  m_nominal_value=1  T_specify=off  T_priority=High  T=300 K  T_nominal_specify=off  T_nominal_unit=K  T_nominal_value=1  Q_specify=off  Q_priority=None  Q=0 W  Q_nominal_specify=off  Q_nominal_unit=W  Q_nominal_value=1
  muur_4_hout1 : fl_lib/Thermal/Thermal Elements/Thermal Mass  mass_type=foundation.enum.constant_variable.constant  mass=sauna2_muur_4_hout_2_m kg  sp_heat=cp_poplar J/(K*kg)  mass_min=1e-6 kg  num_ports=foundation.enum.numPorts2.one  m_specify=off  m_priority=High  m=1 kg  m_nominal_specify=off  m_nominal_unit=kg  m_nominal_value=1  T_specify=off  T_priority=High  T=300 K  T_nominal_specify=off  T_nominal_unit=K  T_nominal_value=1  Q_specify=off  Q_priority=None  Q=0 W  Q_nominal_specify=off  Q_nominal_unit=W  Q_nominal_value=1
  muur_4_hout_2 : fl_lib/Thermal/Thermal Elements/Thermal Mass  mass_type=foundation.enum.constant_variable.constant  mass=sauna2_muur_4_hout_1_m kg  sp_heat=cp_poplar J/(K*kg)  mass_min=1e-6 kg  num_ports=foundation.enum.numPorts2.one  m_specify=off  m_priority=High  m=1 kg  m_nominal_specify=off  m_nominal_unit=kg  m_nominal_value=1  T_specify=off  T_priority=High  T=300 K  T_nominal_specify=off  T_nominal_unit=K  T_nominal_value=1  Q_specify=off  Q_priority=None  Q=0 W  Q_nominal_specify=off  Q_nominal_unit=W  Q_nominal_value=1
  muur_4_isol1 : fl_lib/Thermal/Thermal Elements/Thermal Mass  mass_type=foundation.enum.constant_variable.constant  mass=sauna2_muur_4_isol_m kg  sp_heat=cp_isol J/(K*kg)  mass_min=1e-6 kg  num_ports=foundation.enum.numPorts2.one  m_specify=off  m_priority=High  m=1 kg  m_nominal_specify=off  m_nominal_unit=kg  m_nominal_value=1  T_specify=off  T_priority=High  T=300 K  T_nominal_specify=off  T_nominal_unit=K  T_nominal_value=1  Q_specify=off  Q_priority=None  Q=0 W  Q_nominal_specify=off  Q_nominal_unit=W  Q_nominal_value=1
  plafond_hout1 : fl_lib/Thermal/Thermal Elements/Thermal Mass  mass_type=foundation.enum.constant_variable.constant  mass=sauna2_plafond_hout_2_m kg  sp_heat=cp_poplar J/(K*kg)  mass_min=1e-6 kg  num_ports=foundation.enum.numPorts2.one  m_specify=off  m_priority=High  m=1 kg  m_nominal_specify=off  m_nominal_unit=kg  m_nominal_value=1  T_specify=off  T_priority=High  T=300 K  T_nominal_specify=off  T_nominal_unit=K  T_nominal_value=1  Q_specify=off  Q_priority=None  Q=0 W  Q_nominal_specify=off  Q_nominal_unit=W  Q_nominal_value=1
  plafond_hout_2 : fl_lib/Thermal/Thermal Elements/Thermal Mass  mass_type=foundation.enum.constant_variable.constant  mass=sauna2_plafond_hout_1_m kg  sp_heat=cp_poplar J/(K*kg)  mass_min=1e-6 kg  num_ports=foundation.enum.numPorts2.one  m_specify=off  m_priority=High  m=1 kg  m_nominal_specify=off  m_nominal_unit=kg  m_nominal_value=1  T_specify=off  T_priority=High  T=300 K  T_nominal_specify=off  T_nominal_unit=K  T_nominal_value=1  Q_specify=off  Q_priority=None  Q=0 W  Q_nominal_specify=off  Q_nominal_unit=W  Q_nominal_value=1
  plafond_isol1 : fl_lib/Thermal/Thermal Elements/Thermal Mass  mass_type=foundation.enum.constant_variable.constant  mass=sauna2_plafond_isol_m kg  sp_heat=cp_isol J/(K*kg)  mass_min=1e-6 kg  num_ports=foundation.enum.numPorts2.one  m_specify=off  m_priority=High  m=1 kg  m_nominal_specify=off  m_nominal_unit=kg  m_nominal_value=1  T_specify=off  T_priority=High  T=300 K  T_nominal_specify=off  T_nominal_unit=K  T_nominal_value=1  Q_specify=off  Q_priority=None  Q=0 W  Q_nominal_specify=off  Q_nominal_unit=W  Q_nominal_value=1
  Heater : PMIOPort  Tag=PMCPort  Side=Left
  Air temperature : Outport
  wires:
  PS-Simulink Converter/1 -> Air temperature/1, Scope/1
  connections:
  Temperature Sensor/RConn2 -- PS-Simulink Converter/LConn1
  Heater/RConn1 -- Lucht/LConn1 -- Temperature Sensor/LConn1 -- Convective Heat Transfer13/LConn1 -- Convective Heat Transfer3/LConn1 -- Convective Heat Transfer1/LConn1 -- Convective Heat Transfer6/LConn1 -- Convective Heat Transfer5/LConn1 -- Convective Heat Transfer9/LConn1 -- Convective Heat Transfer11/LConn1 -- Solver Configuration/RConn1
  Temperature Sensor/RConn1 -- Thermal Reference1/LConn1
  Conductive Heat Transfer24/RConn1 -- muur_2_hout9/LConn1 -- Conductive Heat Transfer25/LConn1
  Conductive Heat Transfer26/RConn1 -- muur_2_hout10/LConn1 -- Conductive Heat Transfer29/LConn1
  Conductive Heat Transfer27/RConn1 -- muur_2_isol4/LConn1 -- Conductive Heat Transfer28/LConn1
  Conductive Heat Transfer30/RConn1 -- muur_2_gips4/LConn1 -- Conductive Heat Transfer31/LConn1
  Convective Heat Transfer7/LConn1 -- Conductive Heat Transfer31/RConn1
  Conductive Heat Transfer27/LConn1 -- Conductive Heat Transfer25/RConn1
  Conductive Heat Transfer30/LConn1 -- Conductive Heat Transfer29/RConn1
  Conductive Heat Transfer28/RConn1 -- Conductive Heat Transfer26/LConn1
  Conductive Heat Transfer24/LConn1 -- Convective Heat Transfer6/RConn1
  Temperature Source3/LConn1 -- Convective Heat Transfer10/RConn1 -- Convective Heat Transfer8/RConn1 -- Convective Heat Transfer4/RConn1 -- Convective Heat Transfer7/RConn1 -- Convective Heat Transfer2/RConn1
  Convective Heat Transfer1/RConn1 -- Conductive Heat Transfer1/LConn1
  Conductive Heat Transfer1/RConn1 -- Conductive Heat Transfer2/LConn1 -- muur 1_hout3/LConn1
  Conductive Heat Transfer3/LConn1 -- Conductive Heat Transfer2/RConn1
  Conductive Heat Transfer3/RConn1 -- Conductive Heat Transfer5/LConn1 -- muur 1_isol1/LConn1
  Conductive Heat Transfer5/RConn1 -- Conductive Heat Transfer4/LConn1
  Conductive Heat Transfer4/RConn1 -- Conductive Heat Transfer6/LConn1 -- muur 1_hout4/LConn1
  Conductive Heat Transfer6/RConn1 -- Convective Heat Transfer2/LConn1
  muur_3_gips2/LConn1 -- Conductive Heat Transfer13/RConn1 -- Conductive Heat Transfer14/LConn1
  Conductive Heat Transfer14/RConn1 -- Convective Heat Transfer4/LConn1
  Conductive Heat Transfer9/RConn1 -- muur_3_hout4/LConn1 -- Conductive Heat Transfer12/LConn1
  Conductive Heat Transfer12/RConn1 -- Conductive Heat Transfer13/LConn1
  Conductive Heat Transfer11/RConn1 -- Conductive Heat Transfer9/LConn1
  Conductive Heat Transfer11/LConn1 -- muur_3_isol1/LConn1 -- Conductive Heat Transfer10/RConn1
  Conductive Heat Transfer8/RConn1 -- Conductive Heat Transfer10/LConn1
  Conductive Heat Transfer8/LConn1 -- muur_3_hout3/LConn1 -- Conductive Heat Transfer7/RConn1
  Conductive Heat Transfer7/LConn1 -- Convective Heat Transfer3/RConn1
  Conductive Heat Transfer16/RConn1 -- Conductive Heat Transfer15/LConn1 -- muur 3_raam1/LConn1
  Conductive Heat Transfer16/LConn1 -- Convective Heat Transfer5/RConn1
  Convective Heat Transfer8/LConn1 -- Conductive Heat Transfer15/RConn1
  Conductive Heat Transfer22/LConn1 -- plafond_hout1/LConn1 -- Conductive Heat Transfer20/RConn1
  Convective Heat Transfer10/LConn1 -- Conductive Heat Transfer22/RConn1
  Conductive Heat Transfer21/RConn1 -- Conductive Heat Transfer20/LConn1
  plafond_isol1/LConn1 -- Conductive Heat Transfer19/RConn1 -- Conductive Heat Transfer21/LConn1
  Conductive Heat Transfer19/LConn1 -- Conductive Heat Transfer18/RConn1
  Conductive Heat Transfer18/LConn1 -- Conductive Heat Transfer17/RConn1 -- plafond_hout_2/LConn1
  Conductive Heat Transfer17/LConn1 -- Convective Heat Transfer9/RConn1
  Conductive Heat Transfer36/RConn1 -- muur_4_hout_2/LConn1 -- Conductive Heat Transfer37/LConn1
  Conductive Heat Transfer37/RConn1 -- Conductive Heat Transfer23/LConn1
  Conductive Heat Transfer23/RConn1 -- muur_4_isol1/LConn1 -- Conductive Heat Transfer32/LConn1
  Conductive Heat Transfer38/RConn1 -- muur_4_hout1/LConn1 -- Conductive Heat Transfer33/LConn1
  Conductive Heat Transfer34/LConn1 -- Conductive Heat Transfer33/RConn1
  Conductive Heat Transfer34/RConn1 -- muur_4_gips1/LConn1 -- Conductive Heat Transfer35/LConn1
  Conductive Heat Transfer35/RConn1 -- Convective Heat Transfer12/LConn1
  Conductive Heat Transfer38/LConn1 -- Conductive Heat Transfer32/RConn1
  Conductive Heat Transfer36/LConn1 -- Convective Heat Transfer11/RConn1
  Convective Heat Transfer12/RConn1 -- Temperature Source2/LConn1 -- Convective Heat Transfer14/RConn1
  Conductive Heat Transfer40/LConn1 -- Convective Heat Transfer13/RConn1
  Conductive Heat Transfer40/RConn1 -- Conductive Heat Transfer39/LConn1 -- muur 4_raam1/LConn1
  Conductive Heat Transfer39/RConn1 -- Convective Heat Transfer14/LConn1

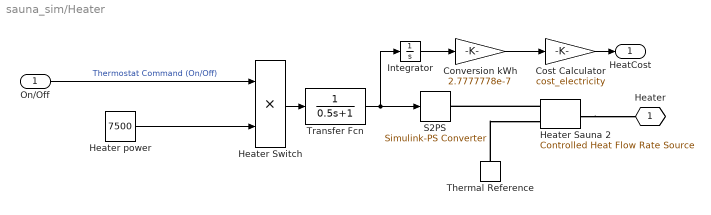
== system sauna_sim/Heater ==
  On/Off : Inport
  Conversion kWh : Gain  Gain=2.7777778e-7  SaturateOnIntegerOverflow=on  OutDataTypeStr=Inherit: Same as input  ParamDataTypeStr=Inherit: Same as input
  Cost Calculator : Gain  Gain=cost_electricity  SaturateOnIntegerOverflow=on  OutDataTypeStr=Inherit: Same as input  ParamDataTypeStr=Inherit: Same as input
  Heater Sauna 2 : fl_lib/Thermal/Thermal Sources/Controlled Heat Flow Rate Source
  Heater Switch : Product  RndMeth=Zero
  Heater power : Constant  Value=7500
  Integrator : Integrator
  S2PS : nesl_utility/Simulink-PS Converter  PhysicalDomain=network_engine_domain  SubClassName=ps_input  LeftPortType=input  RightPortType=output  PseudoPeriodic=off  Frequencies=[]  NoiseDistribution=none  NoiseParameters=[]  Unit=1  AffineConversion=off  FilteringAndDerivatives=zero  SimscapeFilterOrder=1  InputFilterTimeConstant=.001  UdotUserProvided=0
  Thermal Reference : fl_lib/Thermal/Thermal Elements/Thermal Reference
  Transfer Fcn : TransferFcn  Denominator=[0.5 1]
  Heater : PMIOPort  Tag=PMCPort  Side=Right
  HeatCost : Outport  VectorParamsAs1DForOutWhenUnconnected=off
  wires:
  Cost Calculator/1 -> HeatCost/1
  Heater Switch/1 -> Transfer Fcn/1
  Heater power/1 -> Heater Switch/2
  Integrator/1 -> Conversion kWh/1
  Conversion kWh/1 -> Cost Calculator/1
  Transfer Fcn/1 -> S2PS/1, Integrator/1
  On/Off/1 -> Heater Switch/1  "Thermostat Command (On/Off)"
  connections:
  Heater Sauna 2/RConn1 -- S2PS/RConn1
  Thermal Reference/LConn1 -- Heater Sauna 2/RConn2
  Heater Sauna 2/LConn1 -- Heater/RConn1

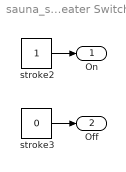
== system sauna_sim/Heater Switch ==
  stroke2 : Constant
  stroke3 : Constant  Value=0
  On : Outport  VectorParamsAs1DForOutWhenUnconnected=off
  Off : Outport  Port=2  VectorParamsAs1DForOutWhenUnconnected=off
  wires:
  stroke2/1 -> On/1
  stroke3/1 -> Off/1

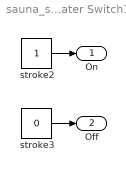
== system sauna_sim/Heater Switch1 ==
  stroke2 : Constant
  stroke3 : Constant  Value=0
  On : Outport  VectorParamsAs1DForOutWhenUnconnected=off
  Off : Outport  Port=2  VectorParamsAs1DForOutWhenUnconnected=off
  wires:
  stroke2/1 -> On/1
  stroke3/1 -> Off/1

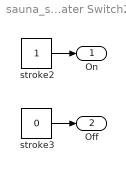
== system sauna_sim/Heater Switch2 ==
  stroke2 : Constant
  stroke3 : Constant  Value=0
  On : Outport  VectorParamsAs1DForOutWhenUnconnected=off
  Off : Outport  Port=2  VectorParamsAs1DForOutWhenUnconnected=off
  wires:
  stroke2/1 -> On/1
  stroke3/1 -> Off/1

== system sauna_sim/Heater Switch3 ==
  stroke2 : Constant
  stroke3 : Constant  Value=0
  On : Outport  VectorParamsAs1DForOutWhenUnconnected=off
  Off : Outport  Port=2  VectorParamsAs1DForOutWhenUnconnected=off
  wires:
  stroke2/1 -> On/1
  stroke3/1 -> Off/1

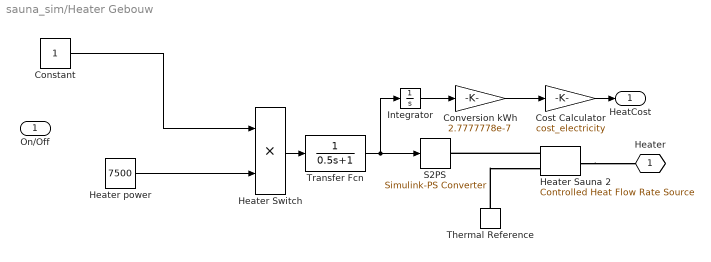
== system sauna_sim/Heater Gebouw ==
  On/Off : Inport
  Constant : Constant
  Conversion kWh : Gain  Gain=2.7777778e-7  SaturateOnIntegerOverflow=on  OutDataTypeStr=Inherit: Same as input  ParamDataTypeStr=Inherit: Same as input
  Cost Calculator : Gain  Gain=cost_electricity  SaturateOnIntegerOverflow=on  OutDataTypeStr=Inherit: Same as input  ParamDataTypeStr=Inherit: Same as input
  Heater Sauna 2 : fl_lib/Thermal/Thermal Sources/Controlled Heat Flow Rate Source
  Heater Switch : Product  RndMeth=Zero
  Heater power : Constant  Value=7500
  Integrator : Integrator
  S2PS : nesl_utility/Simulink-PS Converter  PhysicalDomain=network_engine_domain  SubClassName=ps_input  LeftPortType=input  RightPortType=output  PseudoPeriodic=off  Frequencies=[]  NoiseDistribution=none  NoiseParameters=[]  Unit=1  AffineConversion=off  FilteringAndDerivatives=zero  SimscapeFilterOrder=1  InputFilterTimeConstant=.001  UdotUserProvided=0
  Thermal Reference : fl_lib/Thermal/Thermal Elements/Thermal Reference
  Transfer Fcn : TransferFcn  Denominator=[0.5 1]
  Heater : PMIOPort  Tag=PMCPort  Side=Right
  HeatCost : Outport  VectorParamsAs1DForOutWhenUnconnected=off
  wires:
  Cost Calculator/1 -> HeatCost/1
  Heater Switch/1 -> Transfer Fcn/1
  Heater power/1 -> Heater Switch/2
  Integrator/1 -> Conversion kWh/1
  Conversion kWh/1 -> Cost Calculator/1
  Transfer Fcn/1 -> S2PS/1, Integrator/1
  Constant/1 -> Heater Switch/1
  connections:
  Heater Sauna 2/RConn1 -- S2PS/RConn1
  Thermal Reference/LConn1 -- Heater Sauna 2/RConn2
  Heater Sauna 2/LConn1 -- Heater/RConn1
